simulink library "dspadpt3"  (Simulink 8.2)
settings: Solver=ode45  SolverMode=SingleTasking  StartTime=0.0  StopTime=10.0  RelTol=1e-3
values from neighbouring files (symbols this model uses):
  D = D + B    [rebuffer_delay.m]
undefined symbols (not defined in the file or in its folder): len_measure, len_state, num_cols, num_rows, param, slselsubs
libraries: dspsigattribs x12, dspmtrx3 x2, dspsigops x2, adptfiltsubsys x1, dspsolvers x1
settings Model: RequirementInfo=9  FPTRunName=Active  Creator=don  LastModifiedBy=sconahan  ExtModeAutoUpdateStatusClock=off
settings Model: ForwardingTableString=|
  | ||__slOldName__||dspadpt3/RLS
  | Adaptive Filter||__slNewName__||dspobslib/RLS
  | Adaptive Filter||__slOldName__||dspadpt3/LMS
  | Adaptive Filter||__slNewName__||dspobslib/LMS
  | Adaptive Filter||__slOldName__||dspadpt3/Kalman
  | Adaptive Filter||__slNewName__||dspobslib/Kalman
  | Adaptive Filter

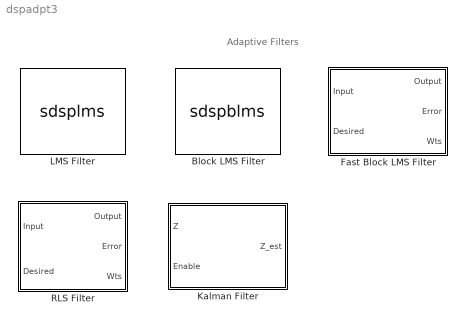
== system dspadpt3 ==
  note: Adaptive Filters
  Block LMS Filter : S-Function  FunctionName=sdspblms  Parameters=L,N,stepflag,mu,leakage,addnparflag,ic,Adapt,resetflag,weights  EnableBusSupport=off  mask(Block LMS Filter){algo=Block LMS, ShowPortLabels=off, L=32, N=32, stepflag=Dialog, mu=0.1, leakage=1.0, addnparflag=on, ic=0, Adapt=off, resetflag=None, weights=on}
      mask prompts: algo "dummy1"; ShowPortLabels "dummy2"; L "Filter length:"; N "Block size:"; stepflag "Specify step size via:"; mu "Step size (mu):"; leakage "Leakage factor (0 to 1):"; addnparflag "dummy3"; ic "Initial value of filter weights:"; Adapt "Adapt port"; resetflag "Reset port:"; weights "Output filter weights"
      mask help:
      | Computes filter weights based on the Block LMS algorithm for filtering of the input signal. The filter weights are updated once for every block of data that is processed.
      |
      | Select the Adapt port check box to create an Adapt port on the block. When the input to this port is nonzero, the block continuously updates the filter weights. When the input to this port is zero, the filter weights remain constant.
      |
      | If the Reset port is enabled and a reset event occurs, the block resets the filter weights to their initial values.
      mask init:
      | resetflag = resetflag-1;
      | [si,so]=dspblkblklms('icon');
      mask Help: eval('blocksethelp');
      mask TypeOptions algo: Block LMS | Fast Block LMS
      mask TypeOptions stepflag: Dialog | Input port
      mask Callback stepflag: dspblkblklms;
      mask TypeOptions resetflag: None | Rising edge | Falling edge | Either edge | Non-zero sample
      mask Display:
      | disp('Block\nLMS')
      | port_label('input',si(1).port, si(1).txt);
      | port_label('input',si(2).port, si(2).txt);
      | port_label('input',si(3).port, si(3).txt);
      | port_label('input',si(4).port, si(4).txt);
      | port_label('input',si(5).port, si(5).txt);
      | 
      | port_label('output',so(1).port, so(1).txt);
      | port_label('output',so(2).port, so(2).txt);
      | port_label('output',so(3).port, so(3).txt);
  Fast Block LMS Filter : Subsystem  mask(Fast Block LMS Filter){algo=Fast Block LMS, L=32, N=32, stepflag=Dialog, mu=0.008, leakage=1.0, addnparflag=on, ic=0, Adapt=off, resetflag=None, weights=on}
      mask prompts: algo "Algorithm:"; L "Filter length:"; N "Block size:"; stepflag "Specify step size via:"; mu "Step size (mu):"; leakage "Leakage factor (0 to 1):"; addnparflag "Dummy parameter"; ic "Initial value of filter weights:"; Adapt "Adapt port"; resetflag "Reset port:"; weights "Output filter weights"
      mask help:
      | Computes filter weights based on the Fast Block LMS algorithm for filtering of the input signal. The filter weights are updated once for every block of data that is processed. This block uses FFT for fast convolution.
      |
      | Select the Adapt port check box to create an Adapt port on the block. When the input to this port is nonzero, the block continuoulsy updates the filter weights. When the input to this port is zero, the filter weights remain constant.
      |
      | If the Reset port is enabled and a reset event occurs, the block resets the filter weights to their initial values.
      mask init:
      | dspblkfblms('init');
      settings: ErrorFcn=dspblkadpterrfcn
      mask Help: eval('blocksethelp');
      mask TypeOptions algo: Block LMS | Fast Block LMS
      mask TypeOptions stepflag: Dialog | Input port
      mask Callback stepflag: dspblkfblms('addparams');
      mask TypeOptions resetflag: None | Rising Edge | Falling Edge | Either Edge | Non-zero sample
      mask Display: disp('Fast Block\nLMS');
  Kalman Filter : Subsystem  DialogController=dspDDGCreate  DialogControllerArgs=DataTag0  mask(Kalman Filter){num_targets=10, sourceEnable=Specify via input port <Enable>, isReset=on, X=zeros([6, 1]), P=10*eye(6), A=[1 0 1 0 0 0;0 1 0 1 0 0; 0 0 1 0 0 0; 0 0 0 1 0 0; 0 0 0 0 1 0; 0 0 0 0 0 1], sourceMeasure=Specify via Dialog, H=[1 0 0 0 0 0; 0 1 0 0 0 0; 0 0 0 0 1 0; 0 0 0 0 0 1], Q=0.05*eye(6), R=eye(4), isOutputEstMeasure=on, isOutputEstState=off, isOutputEstError=off, isOutputPrdMeasure=off, isOutputPrdState=off, isOutputPrdError=off}
      mask prompts: num_targets "Number of filters:"; sourceEnable "Enable filters:"; isReset "Reset estimated state and estimated error covariance when filters are disabled"; X "Initial condition for state:"; P "Initial condition for estimation error covariance:"; A "State transition matrix:"; sourceMeasure "Measurement matrix source:"; H "Measurement matrix:"; Q "Process noise covariance:"; R "Measurement noise covariance:"; isOutputEstMeasure "Output updated measurement"; isOutputEstState "Output updated state"; isOutputEstError "Output updated estimation error"; isOutputPrdMeasure "Output predicted measurement"; isOutputPrdState "Output predicted state"; isOutputPrdError "Output predicted estimation error"
      mask help:
      | Estimate the state of a dynamic system from a series of incomplete and/or noisy measurements. This block can use the previously estimated state to predict the current state. It can also use the current measurement and the predicted state to estimate the current state value.
      |
      | All filters have the same state transition matrix, measurement matrix, initial conditions, and noise covariance, but their state, measurement, enable, and MSE signals are unique. Within the state, measurement, enable, and MSE signals, each column corresponds to a filter.
      mask init:
      | blkh = gcbh;
      | [len_state,len_measure,param] = deal(1,1,[]);
      | % Check for the presence of at least one output port and reconfigure block based on control parameters
      | errmsg = dspblkkalman('init',blkh,sourceEnable,isReset,sourceMeasure,isOutputEstMeasure,isOutputEstState,isOutputEstError,isOutputPrdMeasure,isOutputPrdState,isOutputPrdError);
      | % Get names for existing ports
      | [inport,outport] = dspblkkalman('icon', blkh);
      | if isempty(errmsg)
      |     % Check remaining parameters. Some checking was already done, by the dialog callback and by the above call to dspblkkalman.
      |     [errmsg,num_targets,len_state,len_measure,param] = dspblkkalman('check_param',blkh,true,sourceMeasure,num_targets,A,H,X,P,R,Q);
      | end
      | if ~isempty(errmsg)
      |     error(errmsg);
      | end
      mask Help: eval('blocksethelp');
      mask TypeOptions sourceEnable: Always | Specify via input port <Enable>
      mask TypeOptions sourceMeasure: Specify via Dialog | Input port <H>
      mask Display:
      | disp('Kalman\nFilter');
      | port_label('input',1, 'Z');
      | port_label('input',inport(1).port, inport(1).txt);
      | port_label('input',inport(2).port, inport(2).txt);
      | port_label('output',outport(1).port, outport(1).txt);
      | port_label('output',outport(2).port, outport(2).txt);
      | port_label('output',outport(3).port, outport(3).txt);
      | port_label('output',outport(4).port, outport(4).txt);
      | port_label('output',outport(5).port, outport(5).txt);
      | port_label('output',outport(6).port, outport(6).txt);
  LMS Filter : S-Function  DialogController=dspDDGCreate  DialogControllerArgs=DataTag1  FunctionName=sdsplms  Parameters=Algo,L,stepflag,mu,leakage,ic,Adapt,resetflag,weights,dtInfo.firstCoeffMode,dtInfo.firstCoeffWordLength,dtInfo.firstCoeffFracLength,dtInfo.secondCoeffMode,dtInfo.secondCoeffWordLength,dtInfo.secondCoeffFracLength,dtInfo.prodOutputMode,dtInfo.prodOutputWordLength,dtInfo.prodOutputFracLength,dtInfo.prodOutput2Mode,dtInfo.prodOutput2WordLength,dtInfo.prodOutput2FracLength,dtInfo.prodOutput3Mode,dtInfo.prodOutput3WordLength,dtInfo.prodOutput3FracLength,dtInfo.prodOutput4Mode,dtInfo.prodOutput4WordLength,dtInfo.prodOutput4FracLength,dtInfo.quotientMode,dtInfo.quotientWordLength,dtInfo.quotientFracLength,dtInfo.accumMode,dtInfo.accumWordLength,dtInfo.accumFracLength,dtInfo.accum2Mode,dtInfo.accum2WordLength,dtInfo.accum2FracLength,dtInfo.memoryMode,dtInfo.memoryWordLength,dtInfo.memoryFracLength,dtInfo.roundingMode,dtInfo.overflowMode  EnableBusSupport=off  mask(LMS Filter){ShowPortLabels=off, Algo=LMS, L=32, stepflag=Dialog, mu=0.1, leakage=1.0, ic=0, Adapt=off, resetflag=None, weights=on, firstCoeffMode=Same word length as first input, firstCoeffWordLength=16, firstCoeffFracLength=15, secondCoeffMode=User-defined, secondCoeffWordLength=2, secondCoeffFracLength=15, accumMode=Same as first input, accumWordLength=32, accumFracLength=20, accum2Mode=User-defined, accum2FracLength=20, prodOutputMode=Same as first input, prodOutputWordLength=32, prodOutputFracLength=20, prodOutput2Mode=User-defined, prodOutput2FracLength=20, prodOutput3Mode=User-defined, prodOutput3FracLength=20, prodOutput4Mode=User-defined, prodOutput4FracLength=20, quotientMode=User-defined, quotientFracLength=20, memoryMode=Same as first input, memoryWordLength=16, memoryFracLength=15, roundingMode=Floor, overflowMode=off, addnparflag=off, LockScale=off}
      mask prompts: ShowPortLabels "dummy"; Algo "Algorithm:"; L "Filter length:"; stepflag "Specify step size via:"; mu "Step size (mu):"; leakage "Leakage factor (0 to 1):"; ic "Initial value of filter weights:"; Adapt "Adapt port"; resetflag "Reset port:"; weights "Output filter weights"; firstCoeffMode "Step size (mu) attributes:"; firstCoeffWordLength "Step size (mu) word length:"; firstCoeffFracLength "Step size (mu) fraction length:"; secondCoeffMode "Leakage factor attributes:"; secondCoeffWordLength "DUMMY lkg wordlength:"; secondCoeffFracLength "Leakage factor fraction length:"; accumMode "Accumulator (XTX) attributes:"; accumWordLength "Accumulator (XTX) word length:"; accumFracLength "Accumulator (XTX) fraction length:"; accum2Mode "Accumulator (WTX) attributes:"; accum2FracLength "Accumulator (WTX) fraction length:"; prodOutputMode "Product (XTX) output attributes:"; prodOutputWordLength "Product (XTX) output word length:"; prodOutputFracLength "Product (XTX) output fraction length:"; prodOutput2Mode "Product (WTX) output attributes:"; prodOutput2FracLength "Product (WTX) output fraction length:"; prodOutput3Mode "Product (mu*e) output attributes:"; prodOutput3FracLength "Product (mu*e) output fraction length:"; prodOutput4Mode "Product (Q*x) output attributes:"; prodOutput4FracLength "Product (Q*x) output fraction length:"; quotientMode "Quotient attributes:"; quotientFracLength "Quotient fraction length:"; memoryMode "State memory attributes:"; memoryWordLength "State memory word length:"; memoryFracLength "State memory fraction length:"; roundingMode "Round integer calculations toward:"; overflowMode "Saturate on integer overflow"; addnparflag "Dummy parameter"; LockScale "Lock scaling"
      mask help:
      | Adapts the filter weights based on the chosen algorithm for filtering of the input signal.
      |
      | Select the Adapt port check box to create an Adapt port on the block. When the input to this port is nonzero, the block continuously updates the filter weights. When the input to this port is zero, the filter weights remain constant.
      |
      | If the Reset port is enabled and a reset event occurs, the block resets the filter weights to their initial values.
      mask init:
      | resetflag = resetflag-1;
      | ic        = flipud(ic(:));
      | dtInfo    = dspblkGetLMSFilterDTRowInfo(gcbh);
      | [si,so,disp_str] = dspblklms;
      mask Help: eval('blocksethelp');
      mask TypeOptions Algo: LMS | Normalized LMS | Sign-Error LMS | Sign-Data LMS | Sign-Sign LMS
      mask TypeOptions stepflag: Dialog | Input port
      mask TypeOptions resetflag: None | Rising edge | Falling edge | Either edge | Non-zero sample
      mask TypeOptions firstCoeffMode: Same word length as first input | Specify word length | Binary point scaling | Slope and bias scaling | User-defined
      mask TypeOptions secondCoeffMode: Same word length as first input | Specify word length | Binary point scaling | Slope and bias scaling | User-defined
      mask TypeOptions accumMode: Same as first input | Binary point scaling | Slope and bias scaling | User-defined
      mask TypeOptions accum2Mode: Same as first accumulator | Binary point scaling | Slope and bias scaling | User-defined
      mask TypeOptions prodOutputMode: Same as first input | Binary point scaling | Slope and bias scaling | User-defined
      mask TypeOptions prodOutput2Mode: Same as first product | Binary point scaling | Slope and bias scaling | User-defined
      mask TypeOptions prodOutput3Mode: Same as first product | Binary point scaling | Slope and bias scaling | User-defined
      mask TypeOptions prodOutput4Mode: Same as first product | Binary point scaling | Slope and bias scaling | User-defined
      mask TypeOptions quotientMode: Same as first product | Binary point scaling | Slope and bias scaling | User-defined
      mask TypeOptions memoryMode: Same as first input | Binary point scaling | Slope and bias scaling | User-defined
      mask TypeOptions roundingMode: Ceiling | Convergent | Floor | Nearest | Round | Simplest | Zero
      mask Display:
      | disp(disp_str)
      | port_label('input',si(1).port, si(1).txt);
      | port_label('input',si(2).port, si(2).txt);
      | port_label('input',si(3).port, si(3).txt);
      | port_label('input',si(4).port, si(4).txt);
      | port_label('input',si(5).port, si(5).txt);
      | 
      | port_label('output',so(1).port, so(1).txt);
      | port_label('output',so(2).port, so(2).txt);
      | port_label('output',so(3).port, so(3).txt);
  RLS Filter : Subsystem  mask(RLS filter){L=32, lambdaflag=Dialog, lambda=1.0, addnparflag=on, ic=0, delta=0.1, Adapt=off, resetflag=None, weights=on}
      mask prompts: L "Filter length:"; lambdaflag "Specify forgetting factor via:"; lambda "Forgetting factor (0 to 1):"; addnparflag "Dummy parameter"; ic "Initial value of filter weights:"; delta "Initial input variance estimate:"; Adapt "Adapt port"; resetflag "Reset port:"; weights "Output filter weights"
      mask help:
      | Computes filter weights based on the exponentially weighted recursive least-squares (RLS) algorithm for adaptive filtering of the input signal.
      |
      | Select the Adapt port check box to create an Adapt port on the block. When the input to this port is nonzero, the block continuoulsy updates the filter weights. When the input to this port is zero, the filter weights remain constant.
      |
      | If the Reset port is enabled and a reset event occurs, the block resets the filter weights to their initial values.
      mask init:
      | dspblkrls('init', L, lambda, ic);
      settings: ErrorFcn=dspblkadpterrfcn
      mask Help: eval('blocksethelp');
      mask TypeOptions lambdaflag: Dialog | Input port
      mask Callback lambdaflag: dspblkrls('addparams');
      mask TypeOptions resetflag: None | Rising edge | Falling edge | Either edge | Non-zero sample
      mask Display: disp('RLS');

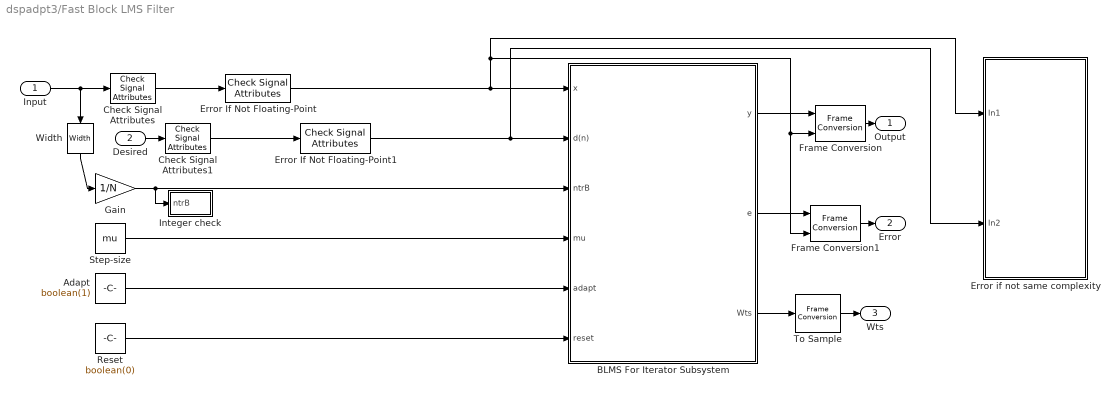
== system dspadpt3/Fast Block LMS Filter ==
  Input : Inport
  Desired : Inport  Port=2
  Adapt : Constant  Value=boolean(1)
  BLMS For Iterator Subsystem : Subsystem  TreatAsAtomicUnit=on  mask{algo_for=Fast Block LMS, stepflag_for=off, weights_for=on}
      mask prompts: algo_for "Algorithm:"; stepflag_for "Input step size via port:"; weights_for "Send filter weights to output:"
      mask init:
      | dspblkfblmsfor;
      mask TypeOptions algo_for: Block LMS | Fast Block LMS
  Check Signal Attributes : dspsigattribs/Check Signal Attributes  SigAttribCheckMethod=Matches attributes exactly  Complexity=Ignore  Frame=Ignore  DimsCheckMethod=Is...  Dimensions=Full matrix (2-D)  DatatypeCheckMethod=Ignore  DatatypeGeneral=Boolean  DtypeFloatSpecific=Any floating-point  DtypeFixedSpecific=Any fixed-point  DtypeIntSpecific=Any integer  SampleMode=Ignore
  Check Signal Attributes1 : dspsigattribs/Check Signal Attributes  SigAttribCheckMethod=Matches attributes exactly  Complexity=Ignore  Frame=Ignore  DimsCheckMethod=Is...  Dimensions=Full matrix (2-D)  DatatypeCheckMethod=Ignore  DatatypeGeneral=Boolean  DtypeFloatSpecific=Any floating-point  DtypeFixedSpecific=Any fixed-point  DtypeIntSpecific=Any integer  SampleMode=Ignore
  Error If Not Floating-Point : dspsigattribs/Check Signal Attributes  SigAttribCheckMethod=Does not match attributes exactly  Complexity=Ignore  Frame=Ignore  DimsCheckMethod=Ignore  Dimensions=1-D  DatatypeCheckMethod=Is...  DatatypeGeneral=Floating-point  DtypeFloatSpecific=Any floating-point  DtypeFixedSpecific=Any fixed-point  DtypeIntSpecific=Any integer  SampleMode=Ignore
  Error If Not Floating-Point1 : dspsigattribs/Check Signal Attributes  SigAttribCheckMethod=Does not match attributes exactly  Complexity=Ignore  Frame=Ignore  DimsCheckMethod=Ignore  Dimensions=1-D  DatatypeCheckMethod=Is...  DatatypeGeneral=Floating-point  DtypeFloatSpecific=Any floating-point  DtypeFixedSpecific=Any fixed-point  DtypeIntSpecific=Any integer  SampleMode=Ignore
  Error if not same complexity : Subsystem  TreatAsAtomicUnit=on  SimViewingDevice=on
  Frame Conversion : FrameConversion  InheritSamplingMode=on
  Frame Conversion1 : FrameConversion  InheritSamplingMode=on
  Gain : Gain  Gain=1/N  SaturateOnIntegerOverflow=on  OutDataTypeStr=Inherit: Same as input  ParamDataTypeStr=Inherit: Same as input
  Integer check : Subsystem
  Reset : Constant  Value=boolean(0)
  Step-size : Constant  Value=mu  OutDataTypeStr=Inherit: Inherit via back propagation
  To Sample : FrameConversion  OutFrame=Sample-based
  Width : Width
  Output : Outport
  Error : Outport  Port=2
  Wts : Outport  Port=3
  wires:
  Step-size/1 -> BLMS For Iterator Subsystem/4(mu)
  To Sample/1 -> Wts/1
  BLMS For Iterator Subsystem/3(Wts) -> To Sample/1
  Desired/1 -> Check Signal Attributes1/1
  Input/1 -> Width/1, Check Signal Attributes/1
  Gain/1 -> Integer check/1(ntrB), BLMS For Iterator Subsystem/3(ntrB)
  Width/1 -> Gain/1
  Reset/1 -> BLMS For Iterator Subsystem/6(reset)
  Adapt/1 -> BLMS For Iterator Subsystem/5(adapt)
  BLMS For Iterator Subsystem/1(y) -> Frame Conversion/1
  Frame Conversion/1 -> Output/1
  BLMS For Iterator Subsystem/2(e) -> Frame Conversion1/1
  Frame Conversion1/1 -> Error/1
  Error If Not Floating-Point/1 -> Frame Conversion/2, Frame Conversion1/2, Error if not same complexity/1(In1), BLMS For Iterator Subsystem/1(x)
  Error If Not Floating-Point1/1 -> Error if not same complexity/2(In2), BLMS For Iterator Subsystem/2(d(n))
  Check Signal Attributes1/1 -> Error If Not Floating-Point1/1
  Check Signal Attributes/1 -> Error If Not Floating-Point/1

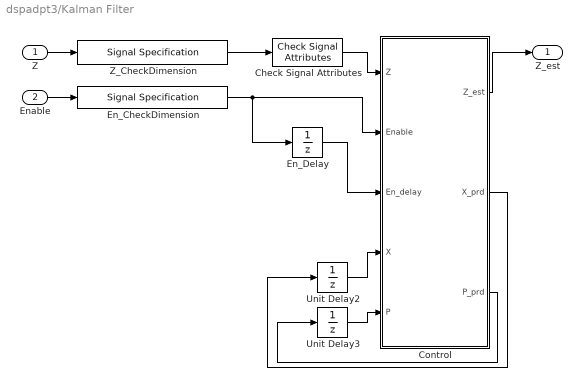
== system dspadpt3/Kalman Filter ==
  Z : Inport
  Enable : Inport  Port=2
  Check Signal Attributes : dspsigattribs/Check Signal Attributes  SigAttribCheckMethod=Does not match attributes exactly  Complexity=Real  Frame=Ignore  DimsCheckMethod=Ignore  Dimensions=Scalar (1-D or 2-D)  DatatypeCheckMethod=Is...  DatatypeGeneral=Floating-point  DtypeFloatSpecific=Any floating-point  DtypeFixedSpecific=Any fixed-point  DtypeIntSpecific=Any integer  SampleMode=Ignore
  Control : Subsystem
  En_CheckDimension : SignalSpecification  Dimensions=[1, num_targets]
  En_Delay : UnitDelay  SampleTime=-1
  Unit Delay2 : UnitDelay  InitialCondition=param.XAll  SampleTime=-1
  Unit Delay3 : UnitDelay  InitialCondition=param.PAll  SampleTime=-1
  Z_CheckDimension : SignalSpecification  Dimensions=[len_measure, num_targets]
  Z_est : Outport
  wires:
  Unit Delay2/1 -> Control/4(X)
  Unit Delay3/1 -> Control/5(P)
  Z_CheckDimension/1 -> Check Signal Attributes/1
  Z/1 -> Z_CheckDimension/1
  Control/1(Z_est) -> Z_est/1
  Check Signal Attributes/1 -> Control/1(Z)
  Control/2(X_prd) -> Unit Delay2/1
  Control/3(P_prd) -> Unit Delay3/1
  Enable/1 -> En_CheckDimension/1
  En_CheckDimension/1 -> En_Delay/1, Control/2(Enable)
  En_Delay/1 -> Control/3(En_delay)

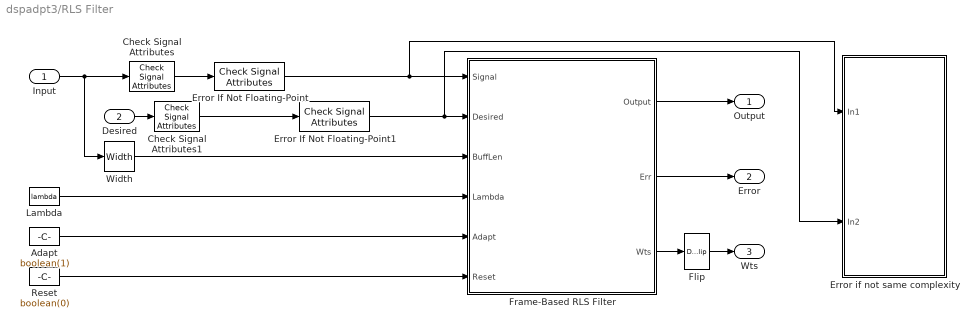
== system dspadpt3/RLS Filter ==
  Input : Inport
  Desired : Inport  Port=2
  Adapt : Constant  Value=boolean(1)
  Check Signal Attributes : dspsigattribs/Check Signal Attributes  SigAttribCheckMethod=Matches attributes exactly  Complexity=Ignore  Frame=Ignore  DimsCheckMethod=Is...  Dimensions=Full matrix (2-D)  DatatypeCheckMethod=Ignore  DatatypeGeneral=Boolean  DtypeFloatSpecific=Any floating-point  DtypeFixedSpecific=Any fixed-point  DtypeIntSpecific=Any integer  SampleMode=Ignore
  Check Signal Attributes1 : dspsigattribs/Check Signal Attributes  SigAttribCheckMethod=Matches attributes exactly  Complexity=Ignore  Frame=Ignore  DimsCheckMethod=Is...  Dimensions=Full matrix (2-D)  DatatypeCheckMethod=Ignore  DatatypeGeneral=Boolean  DtypeFloatSpecific=Any floating-point  DtypeFixedSpecific=Any fixed-point  DtypeIntSpecific=Any integer  SampleMode=Ignore
  Error If Not Floating-Point : dspsigattribs/Check Signal Attributes  SigAttribCheckMethod=Does not match attributes exactly  Complexity=Ignore  Frame=Ignore  DimsCheckMethod=Ignore  Dimensions=1-D  DatatypeCheckMethod=Is...  DatatypeGeneral=Floating-point  DtypeFloatSpecific=Any floating-point  DtypeFixedSpecific=Any fixed-point  DtypeIntSpecific=Any integer  SampleMode=Ignore
  Error If Not Floating-Point1 : dspsigattribs/Check Signal Attributes  SigAttribCheckMethod=Does not match attributes exactly  Complexity=Ignore  Frame=Ignore  DimsCheckMethod=Ignore  Dimensions=1-D  DatatypeCheckMethod=Is...  DatatypeGeneral=Floating-point  DtypeFloatSpecific=Any floating-point  DtypeFixedSpecific=Any fixed-point  DtypeIntSpecific=Any integer  SampleMode=Ignore
  Error if not same complexity : Subsystem  TreatAsAtomicUnit=on  SimViewingDevice=on
  Flip : DSPFlip
  Frame-Based RLS Filter : Subsystem  TreatAsAtomicUnit=on  mask{weights_for=on}
      mask prompts: weights_for "Send filter weights to output:"
      mask init:
      | dspblkrlsfor;
  Lambda : Constant  Value=lambda  OutDataTypeStr=Inherit: Inherit via back propagation
  Reset : Constant  Value=boolean(0)
  Width : Width
  Output : Outport
  Error : Outport  Port=2
  Wts : Outport  Port=3
  wires:
  Check Signal Attributes/1 -> Error If Not Floating-Point/1
  Error If Not Floating-Point1/1 -> Error if not same complexity/2(In2), Frame-Based RLS Filter/2(Desired)
  Error If Not Floating-Point/1 -> Error if not same complexity/1(In1), Frame-Based RLS Filter/1(Signal)
  Check Signal Attributes1/1 -> Error If Not Floating-Point1/1
  Lambda/1 -> Frame-Based RLS Filter/4(Lambda)
  Adapt/1 -> Frame-Based RLS Filter/5(Adapt)
  Width/1 -> Frame-Based RLS Filter/3(BuffLen)
  Input/1 -> Check Signal Attributes/1, Width/1
  Desired/1 -> Check Signal Attributes1/1
  Frame-Based RLS Filter/1(Output) -> Output/1
  Reset/1 -> Frame-Based RLS Filter/6(Reset)
  Frame-Based RLS Filter/2(Err) -> Error/1
  Frame-Based RLS Filter/3(Wts) -> Flip/1
  Flip/1 -> Wts/1

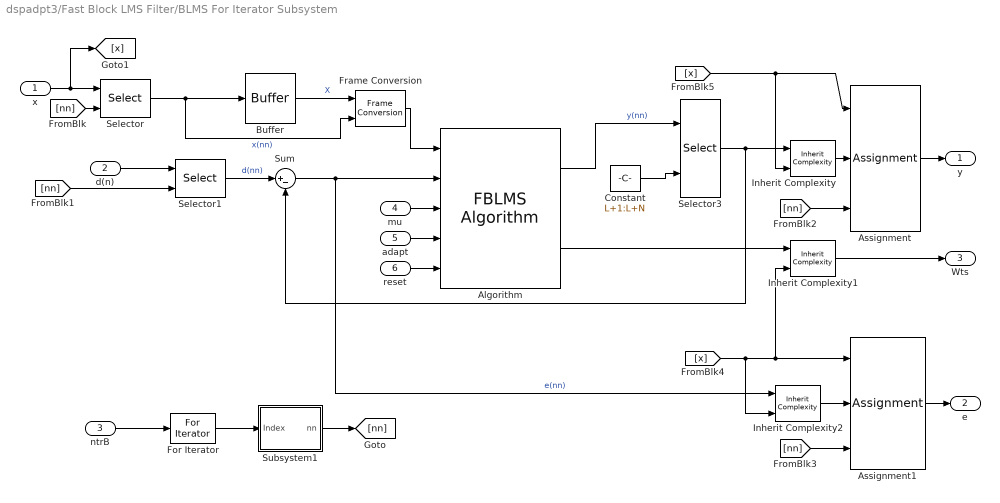
== system dspadpt3/Fast Block LMS Filter/BLMS For Iterator Subsystem ==
  x : Inport
  d(n) : Inport  Port=2
  ntrB : Inport  Port=3
  mu : Inport  Port=4
  adapt : Inport  Port=5
  reset : Inport  Port=6
  Algorithm : adptfiltsubsys/FBLMS Algorithm  weights_algo=on
  Assignment : Assignment  IndexOptions=Index vector (port)  Indices=1  OutputSizes=[1 1]
  Assignment1 : Assignment  IndexOptions=Index vector (port)  Indices=1  OutputSizes=[1 1]
  Buffer : Buffer  N=L+N  V=L  TreatMby1Signals=One channel
  Constant : Constant  Value=L+1:L+N
  For Iterator : ForIterator  IterationSource=external  IterationVariableDataType=double
  Frame Conversion : FrameConversion  InheritSamplingMode=on
  Inherit Complexity : dspsigattribs/Inherit Complexity
  Inherit Complexity1 : dspsigattribs/Inherit Complexity
  Inherit Complexity2 : dspsigattribs/Inherit Complexity
  Selector : Selector  IndexOptions=Index vector (port)  Indices=[1 3]  OutputSizes=1
  Selector1 : Selector  IndexOptions=Index vector (port)  Indices=[1 3]  OutputSizes=1
  Selector3 : Selector  IndexOptions=Index vector (port)  Indices=[1 3]  OutputSizes=1
  Subsystem1 : Subsystem
  Sum : Sum  Inputs=|+-  SaturateOnIntegerOverflow=on
  y : Outport
  e : Outport  Port=2
  Wts : Outport  Port=3
  wires:
  Algorithm/2 -> Inherit Complexity1/1
  adapt/1 -> Algorithm/4
  mu/1 -> Algorithm/3
  Inherit Complexity1/1 -> Wts/1
  Inherit Complexity2/1 -> Assignment1/2
  Inherit Complexity/1 -> Assignment/2
  Sum/1 -> Algorithm/2, Inherit Complexity2/1  "e(nn)"
  Selector1/1 -> Sum/1  "d(nn)"
  [nn] -> Assignment1/3
  Assignment1/1 -> e/1
  ntrB/1 -> For Iterator/1
  For Iterator/1 -> Subsystem1/1(Index)
  Assignment/1 -> y/1
  x/1 -> Selector/1, [x]
  [nn] -> Selector/2
  d(n)/1 -> Selector1/1
  [nn] -> Selector1/2
  Subsystem1/1(nn) -> [nn]
  Selector/1 -> Frame Conversion/2, Buffer/1  "x(nn)"
  reset/1 -> Algorithm/5
  Constant/1 -> Selector3/2
  Selector3/1 -> Sum/2, Inherit Complexity/1
  Algorithm/1 -> Selector3/1  "y(nn)"
  [nn] -> Assignment/3
  [x] -> Inherit Complexity2/2, Assignment1/1, Inherit Complexity1/2
  [x] -> Inherit Complexity/2, Assignment/1
  Buffer/1 -> Frame Conversion/1  "X"
  Frame Conversion/1 -> Algorithm/1

== system dspadpt3/Fast Block LMS Filter/Error if not same complexity ==
  In1 : Inport
  In2 : Inport  Port=2
  Assertion : Assertion  AssertionFailFcn=error('The signals connected to the Input and Desired ports of the Fast Block LMS Filter block must have the same complexity.')
  Probe : Probe  ProbeWidth=off  ProbeSampleTime=off  ProbeComplexityDataType=boolean
  Probe1 : Probe  ProbeWidth=off  ProbeSampleTime=off  ProbeComplexityDataType=boolean
  Relational Operator : RelationalOperator  Operator===  OutDataTypeStr=boolean  ZeroCross=off  InputSameDT=on
  wires:
  Relational Operator/1 -> Assertion/1
  In2/1 -> Probe1/1
  In1/1 -> Probe/1
  Probe1/1 -> Relational Operator/2
  Probe/1 -> Relational Operator/1

== system dspadpt3/Fast Block LMS Filter/Integer check ==
  ntrB : Inport
  Assertion : Assertion  AssertionFailFcn=error('The input frame length is not an integer multiple of the Block length');
  Relational Operator : RelationalOperator  Operator===  OutDataTypeStr=boolean
  Rounding Function : Rounding  Operator=fix
  wires:
  Rounding Function/1 -> Relational Operator/2
  Relational Operator/1 -> Assertion/1
  ntrB/1 -> Relational Operator/1, Rounding Function/1

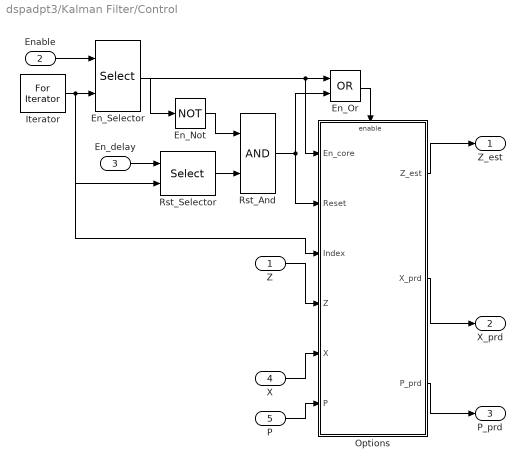
== system dspadpt3/Kalman Filter/Control ==
  Z : Inport
  Enable : Inport  Port=2
  En_delay : Inport  Port=3
  X : Inport  Port=4
  P : Inport  Port=5
  En_Not : Logic  Operator=NOT  AllPortsSameDT=off
  En_Or : Logic  Operator=OR  AllPortsSameDT=off
  En_Selector : Selector  NumberOfDimensions=2  IndexOptions=Select all,Index vector (port)  Indices=-1,1  OutputSizes=1
  Iterator : ForIterator  IterationLimit=num_targets
  Options : Subsystem
  Rst_And : Logic  AllPortsSameDT=off
  Rst_Selector : Selector  NumberOfDimensions=2  IndexOptions=Select all,Index vector (port)  Indices=-1,1  OutputSizes=1
  Z_est : Outport
  X_prd : Outport  Port=2
  P_prd : Outport  Port=3
  wires:
  Iterator/1 -> Options/3(Index), En_Selector/2, Rst_Selector/2
  Options/1(Z_est) -> Z_est/1
  Options/2(X_prd) -> X_prd/1
  Options/3(P_prd) -> P_prd/1
  Z/1 -> Options/4(Z)
  X/1 -> Options/5(X)
  P/1 -> Options/6(P)
  Enable/1 -> En_Selector/1
  En_delay/1 -> Rst_Selector/1
  En_Selector/1 -> En_Not/1, En_Or/1, Options/1(En_core)
  En_Not/1 -> Rst_And/1
  Rst_Selector/1 -> Rst_And/2
  Rst_And/1 -> En_Or/2, Options/2(Reset)
  En_Or/1 -> Options/Enable

== system dspadpt3/RLS Filter/Error if not same complexity ==
  In1 : Inport
  In2 : Inport  Port=2
  Assertion : Assertion  AssertionFailFcn=error('The signals connected to the Input and Desired ports of the RLS Filter block must have the same complexity.')
  Probe : Probe  ProbeWidth=off  ProbeSampleTime=off  ProbeComplexityDataType=boolean
  Probe1 : Probe  ProbeWidth=off  ProbeSampleTime=off  ProbeComplexityDataType=boolean
  Relational Operator : RelationalOperator  Operator===  OutDataTypeStr=boolean  ZeroCross=off  InputSameDT=on
  wires:
  Relational Operator/1 -> Assertion/1
  In2/1 -> Probe1/1
  In1/1 -> Probe/1
  Probe1/1 -> Relational Operator/2
  Probe/1 -> Relational Operator/1

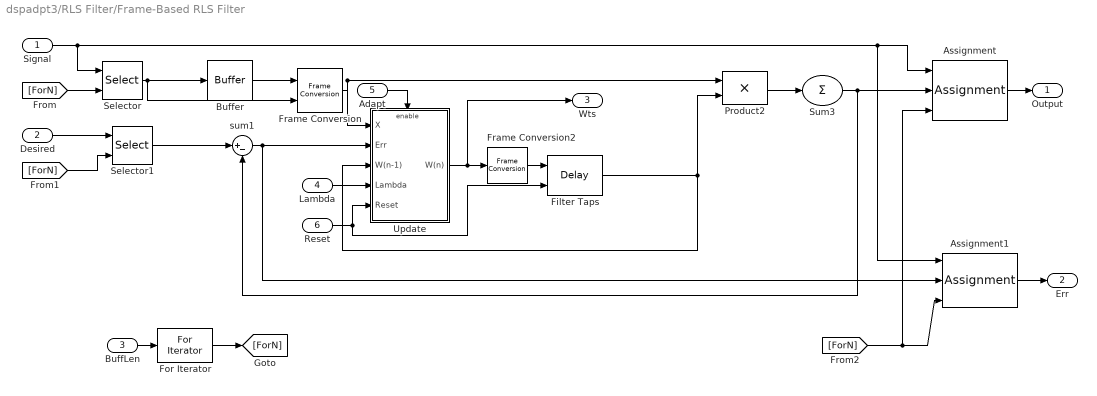
== system dspadpt3/RLS Filter/Frame-Based RLS Filter ==
  Signal : Inport
  Desired : Inport  Port=2
  BuffLen : Inport  Port=3
  Lambda : Inport  Port=4
  Adapt : Inport  Port=5
  Reset : Inport  Port=6
  Assignment : Assignment  IndexOptions=Index vector (port)  Indices=1  OutputSizes=[1 1]
  Assignment1 : Assignment  IndexOptions=Index vector (port)  Indices=1  OutputSizes=[1 1]
  Buffer : Buffer  N=L  V=L-1  TreatMby1Signals=One channel
  Filter Taps : dspsigops/Delay  dly_unit=Samples  delay=1  ic_detail=on  dif_ic_for_ch=off  dif_ic_for_dly=off  ic=flipud(ic(:))  reset_popup=Non-zero sample
  For Iterator : ForIterator  IterationSource=external  IterationLimit=4
  Frame Conversion : FrameConversion  InheritSamplingMode=on
  Frame Conversion2 : FrameConversion  OutFrame=Sample-based
  Product2 : Product  SaturateOnIntegerOverflow=on  OutDataTypeStr=Inherit: Same as first input
  Selector : Selector  IndexOptions=Index vector (port)  Indices=[1 3]  OutputSizes=1
  Selector1 : Selector  IndexOptions=Index vector (port)  Indices=[1 3]  OutputSizes=1
  Sum3 : Sum  Inputs=1  SaturateOnIntegerOverflow=on
  Update : Subsystem
  sum1 : Sum  Inputs=|+-  SaturateOnIntegerOverflow=on  InputSameDT=on  OutDataTypeStr=Inherit: Same as first input
  Output : Outport
  Err : Outport  Port=2
  Wts : Outport  Port=3
  wires:
  Frame Conversion/1 -> Update/1(X), Product2/1
  Lambda/1 -> Update/4(Lambda)
  Adapt/1 -> Update/Enable
  [ForN] -> Assignment1/3, Assignment/3
  Reset/1 -> Update/5(Reset), Filter Taps/2
  sum1/1 -> Assignment1/2, Update/2(Err)
  Sum3/1 -> Assignment/2, sum1/2
  Product2/1 -> Sum3/1
  Update/1(W(n)) -> Wts/1, Frame Conversion2/1
  Buffer/1 -> Frame Conversion/1
  Signal/1 -> Assignment1/1, Assignment/1, Selector/1
  Assignment/1 -> Output/1
  Desired/1 -> Selector1/1
  BuffLen/1 -> For Iterator/1
  Selector/1 -> Frame Conversion/2, Buffer/1
  For Iterator/1 -> [ForN]
  [ForN] -> Selector/2
  [ForN] -> Selector1/2
  Selector1/1 -> sum1/1
  Assignment1/1 -> Err/1
  Frame Conversion2/1 -> Filter Taps/1
  Filter Taps/1 -> Product2/2, Update/3(W(n-1))

== system dspadpt3/Fast Block LMS Filter/BLMS For Iterator Subsystem/Subsystem1 ==
  Index : Inport
  BlkVec : Constant  Value=[1:N]
  Constant : Constant
  Gain : Gain  Gain=N  SaturateOnIntegerOverflow=on  OutDataTypeStr=Inherit: Same as input  ParamDataTypeStr=Inherit: Same as input
  Sum : Sum  Inputs=|+-  SaturateOnIntegerOverflow=on
  Sum1 : Sum  Inputs=|++  SaturateOnIntegerOverflow=on
  nn : Outport
  wires:
  Sum1/1 -> nn/1
  Index/1 -> Sum/1  "n"
  BlkVec/1 -> Sum1/2  "i"
  Gain/1 -> Sum1/1  "(n-1)*N"
  Sum/1 -> Gain/1  "n-1"
  Constant/1 -> Sum/2

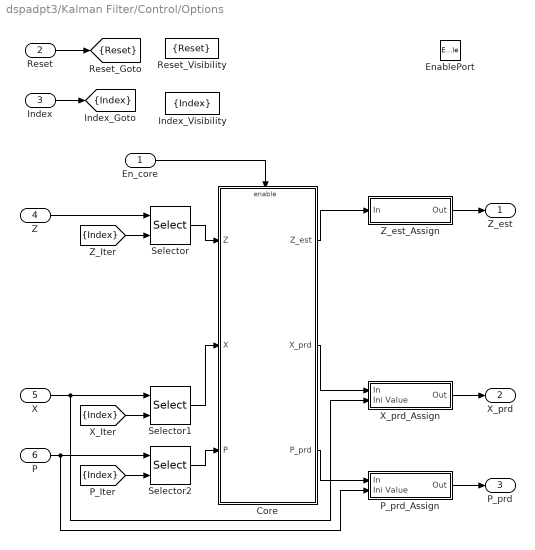
== system dspadpt3/Kalman Filter/Control/Options ==
  En_core : Inport
  Reset : Inport  Port=2
  Index : Inport  Port=3
  Z : Inport  Port=4
  X : Inport  Port=5
  P : Inport  Port=6
  EnablePort : EnablePort
  Core : Subsystem
  Index_Visibility : GotoTagVisibility  GotoTag=Index
  P_prd_Assign : Subsystem
  Reset_Visibility : GotoTagVisibility  GotoTag=Reset
  Selector : Selector  NumberOfDimensions=2  InputPortWidth=3  IndexOptions=Select all,Index vector (port)  Indices=-1,1  OutputSizes=1
  Selector1 : Selector  NumberOfDimensions=2  InputPortWidth=3  IndexOptions=Select all,Index vector (port)  Indices=-1,1  OutputSizes=1
  Selector2 : Selector  NumberOfDimensions=2  InputPortWidth=3  IndexOptions=Select all,Index vector (port)  Indices=-1,1  OutputSizes=1
  X_prd_Assign : Subsystem
  Z_est_Assign : Subsystem  mask{reset_value=zeros(len_measure, 1), num_rows=len_measure, num_cols=num_targets}
      mask prompts: reset_value "Default values:"; num_rows "Number of rows:"; num_cols "Number of Columns:"
      mask Display: disp('Assign/reset')
  Z_est : Outport
  X_prd : Outport  Port=2
  P_prd : Outport  Port=3
  tag scope: Index=scoped, Reset=scoped
  wires:
  Selector/1 -> Core/1(Z)
  X/1 -> Selector1/1, X_prd_Assign/2(Ini Value)
  [Index] -> Selector/2
  [Index] -> Selector2/2
  [Index] -> Selector1/2
  P/1 -> Selector2/1, P_prd_Assign/2(Ini Value)
  Z/1 -> Selector/1
  Selector1/1 -> Core/2(X)
  Selector2/1 -> Core/3(P)
  Core/2(X_prd) -> X_prd_Assign/1(In)
  X_prd_Assign/1(Out) -> X_prd/1
  Core/1(Z_est) -> Z_est_Assign/1(In)
  Core/3(P_prd) -> P_prd_Assign/1(In)
  Z_est_Assign/1(Out) -> Z_est/1
  P_prd_Assign/1(Out) -> P_prd/1
  Index/1 -> [Index]
  Reset/1 -> [Reset]
  En_core/1 -> Core/Enable

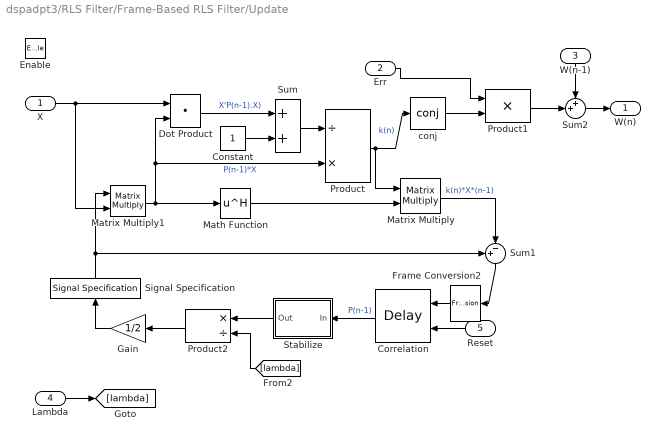
== system dspadpt3/RLS Filter/Frame-Based RLS Filter/Update ==
  X : Inport
  Err : Inport  Port=2
  W(n-1) : Inport  Port=3
  Lambda : Inport  Port=4
  Reset : Inport  Port=5
  Enable : EnablePort
  Constant : Constant  OutDataTypeStr=Inherit: Inherit via back propagation
  Correlation : dspsigops/Delay  dly_unit=Samples  delay=1  ic_detail=on  dif_ic_for_ch=on  dif_ic_for_dly=off  ic=eye(L)./delta  reset_popup=Non-zero sample
  Dot Product : DotProduct  InputSameDT=on  OutDataTypeStr=Inherit: Inherit via internal rule
  Frame Conversion2 : FrameConversion  OutFrame=Sample-based
  Gain : Gain  Gain=1/2  SaturateOnIntegerOverflow=on  OutDataTypeStr=Inherit: Same as input  ParamDataTypeStr=Inherit: Same as input
  Math Function : Math  Operator=hermitian  SaturateOnIntegerOverflow=on
  Matrix Multiply : Product  Multiplication=Matrix(*)
  Matrix Multiply1 : Product  Multiplication=Matrix(*)
  Product : Product  Inputs=/*  SaturateOnIntegerOverflow=on  OutDataTypeStr=Inherit: Same as first input
  Product1 : Product  SaturateOnIntegerOverflow=on  OutDataTypeStr=Inherit: Same as first input
  Product2 : Product  Inputs=*/  SaturateOnIntegerOverflow=on  OutDataTypeStr=Inherit: Same as first input
  Signal Specification : SignalSpecification  Dimensions=[L,L]
  Stabilize : Subsystem
  Sum : Sum  SaturateOnIntegerOverflow=on  OutDataTypeStr=Inherit: Same as first input
  Sum1 : Sum  Inputs=+-|  SaturateOnIntegerOverflow=on
  Sum2 : Sum  Inputs=++|  SaturateOnIntegerOverflow=on
  conj : Math  Operator=conj  SaturateOnIntegerOverflow=on
  W(n) : Outport  InitialOutput=flipud(ic(:))
  wires:
  Constant/1 -> Sum/2
  conj/1 -> Product1/2
  [lambda] -> Product2/2
  Stabilize/1(Out) -> Product2/1
  Product2/1 -> Gain/1
  Lambda/1 -> [lambda]
  Gain/1 -> Signal Specification/1
  Correlation/1 -> Stabilize/1(In)  "P(n-1)"
  Reset/1 -> Correlation/2
  Signal Specification/1 -> Sum1/1, Matrix Multiply1/1
  Sum2/1 -> W(n)/1
  X/1 -> Dot Product/1, Matrix Multiply1/2
  Err/1 -> Product1/1
  W(n-1)/1 -> Sum2/1
  Product1/1 -> Sum2/2
  Sum1/1 -> Frame Conversion2/1
  Matrix Multiply/1 -> Sum1/2  "k(n)*X*(n-1)"
  Math Function/1 -> Matrix Multiply/2
  Product/1 -> Matrix Multiply/1, conj/1  "k(n)"
  Matrix Multiply1/1 -> Dot Product/2, Product/2, Math Function/1  "P(n-1)*X"
  Sum/1 -> Product/1
  Dot Product/1 -> Sum/1  "X'P(n-1).X)"
  Frame Conversion2/1 -> Correlation/1

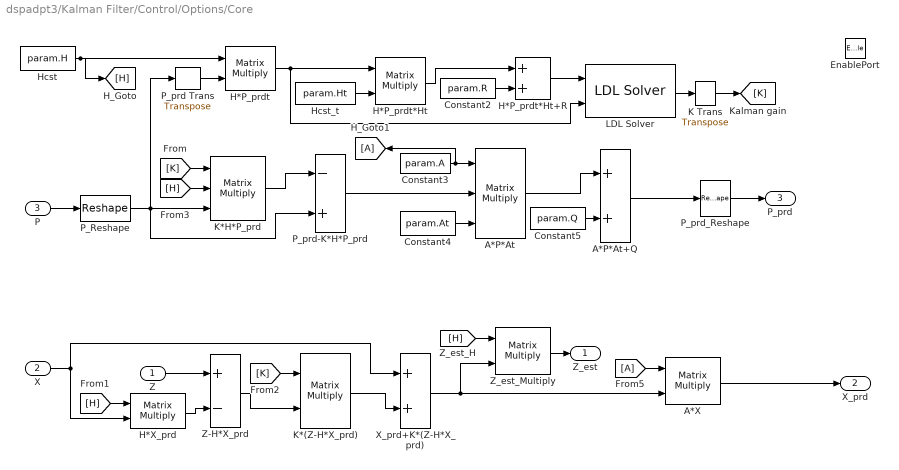
== system dspadpt3/Kalman Filter/Control/Options/Core ==
  Z : Inport
  X : Inport  Port=2
  P : Inport  Port=3
  EnablePort : EnablePort
  A*P*At : Product  Inputs=3  Multiplication=Matrix(*)  OutDataTypeStr=Inherit: Inherit via back propagation  InputSameDT=on
  A*P*At+Q : Sum  OutDataTypeStr=Inherit: Inherit via back propagation  InputSameDT=on
  A*X : Product  Multiplication=Matrix(*)  InputSameDT=on
  Constant2 : Constant  Value=param.R  VectorParams1D=off  OutDataTypeStr=Inherit: Inherit via back propagation
  Constant3 : Constant  Value=param.A  VectorParams1D=off  OutDataTypeStr=Inherit: Inherit via back propagation
  Constant4 : Constant  Value=param.At  VectorParams1D=off  OutDataTypeStr=Inherit: Inherit via back propagation
  Constant5 : Constant  Value=param.Q  VectorParams1D=off  OutDataTypeStr=Inherit: Inherit via back propagation
  H*P_prdt : Product  Multiplication=Matrix(*)  OutDataTypeStr=Inherit: Inherit via back propagation  InputSameDT=on
  H*P_prdt*Ht : Product  Multiplication=Matrix(*)  OutDataTypeStr=Inherit: Inherit via back propagation  InputSameDT=on
  H*P_prdt*Ht+R : Sum  OutDataTypeStr=Inherit: Inherit via back propagation  InputSameDT=on
  H*X_prd : Product  Multiplication=Matrix(*)  OutDataTypeStr=Inherit: Inherit via back propagation  InputSameDT=on
  Hcst : Constant  Value=param.H  VectorParams1D=off  OutDataTypeStr=Inherit: Inherit via back propagation
  Hcst_t : Constant  Value=param.Ht  VectorParams1D=off  OutDataTypeStr=Inherit: Inherit via back propagation
  K Trans : dspmtrx3/Transpose  SystemSampleTime=-1  Hermitian=off  overflowFlag=off
  K*(Z-H*X_prd) : Product  Multiplication=Matrix(*)  InputSameDT=on
  K*H*P_prd : Product  Inputs=3  Multiplication=Matrix(*)  InputSameDT=on  OutDataTypeStr=Inherit: Same as first input
  LDL Solver : dspsolvers/LDL Solver  SystemSampleTime=-1  errmode=Warning
      settings: RTWMemSecFuncInitTerm=Default  RTWMemSecFuncExecute=Default  RTWMemSecDataConstants=Default  RTWMemSecDataInternal=Default  RTWMemSecDataParameters=Default
  P_Reshape : Reshape  OutputDimensionality=Customize  OutputDimensions=[len_state, len_state]
  P_prd Trans : dspmtrx3/Transpose  SystemSampleTime=-1  Hermitian=off  overflowFlag=off
  P_prd-K*H*P_prd : Sum  Inputs=-+  OutDataTypeStr=Inherit: Inherit via back propagation  InputSameDT=on
  P_prd_Reshape : Reshape  OutputDimensionality=Column vector (2-D)
  X_prd+K*(Z-H*X_prd) : Sum  InputSameDT=on
  Z-H*X_prd : Sum  Inputs=+-  InputSameDT=on  OutDataTypeStr=Inherit: Same as first input
  Z_est_Multiply : Product  Multiplication=Matrix(*)  InputSameDT=on
  Z_est : Outport
  X_prd : Outport  Port=2
  P_prd : Outport  Port=3
  wires:
  A*X/1 -> X_prd/1
  A*P*At+Q/1 -> P_prd_Reshape/1
  P_prd-K*H*P_prd/1 -> A*P*At/2
  X/1 -> X_prd+K*(Z-H*X_prd)/1, H*X_prd/2
  P/1 -> P_Reshape/1
  Z-H*X_prd/1 -> K*(Z-H*X_prd)/2
  K*(Z-H*X_prd)/1 -> X_prd+K*(Z-H*X_prd)/2
  H*X_prd/1 -> Z-H*X_prd/2
  [K] -> K*H*P_prd/1
  [H] -> K*H*P_prd/2
  K*H*P_prd/1 -> P_prd-K*H*P_prd/1
  A*P*At/1 -> A*P*At+Q/1
  Constant5/1 -> A*P*At+Q/2
  Constant4/1 -> A*P*At/3
  Constant2/1 -> H*P_prdt*Ht+R/2
  H*P_prdt*Ht/1 -> H*P_prdt*Ht+R/1
  Z/1 -> Z-H*X_prd/1
  [K] -> K*(Z-H*X_prd)/1
  [H] -> H*X_prd/1
  K Trans/1 -> [K]
  P_prd Trans/1 -> H*P_prdt/2
  H*P_prdt/1 -> LDL Solver/2, H*P_prdt*Ht/1
  H*P_prdt*Ht+R/1 -> LDL Solver/1
  LDL Solver/1 -> K Trans/1
  P_prd_Reshape/1 -> P_prd/1
  [H] -> Z_est_Multiply/1
  Z_est_Multiply/1 -> Z_est/1
  X_prd+K*(Z-H*X_prd)/1 -> A*X/2, Z_est_Multiply/2
  [A] -> A*X/1
  Constant3/1 -> A*P*At/1, [A]
  P_Reshape/1 -> K*H*P_prd/3, P_prd-K*H*P_prd/2, P_prd Trans/1
  Hcst/1 -> [H], H*P_prdt/1
  Hcst_t/1 -> H*P_prdt*Ht/2

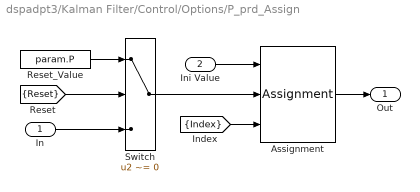
== system dspadpt3/Kalman Filter/Control/Options/P_prd_Assign ==
  In : Inport
  Ini Value : Inport  Port=2
  Assignment : Assignment  NumberOfDimensions=2  IndexOptions=Assign all,Index vector (port)  Indices=-1,1  OutputSizes=slselsubs([num_rows, num_cols],1),slselsubs([num_rows, num_cols],2)
  Reset_Value : Constant  Value=param.P  VectorParams1D=off  OutDataTypeStr=Inherit: Inherit via back propagation
  Switch : Switch  Criteria=u2 ~= 0  SaturateOnIntegerOverflow=on  InputSameDT=on
  Out : Outport
  wires:
  [Index] -> Assignment/3
  Ini Value/1 -> Assignment/1
  Assignment/1 -> Out/1
  Reset_Value/1 -> Switch/1
  [Reset] -> Switch/2
  In/1 -> Switch/3
  Switch/1 -> Assignment/2

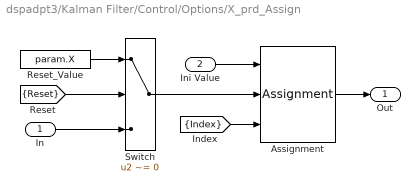
== system dspadpt3/Kalman Filter/Control/Options/X_prd_Assign ==
  In : Inport
  Ini Value : Inport  Port=2
  Assignment : Assignment  NumberOfDimensions=2  IndexOptions=Assign all,Index vector (port)  Indices=-1,1  OutputSizes=slselsubs([num_rows, num_cols],1),slselsubs([num_rows, num_cols],2)
  Reset_Value : Constant  Value=param.X  VectorParams1D=off  OutDataTypeStr=Inherit: Inherit via back propagation
  Switch : Switch  Criteria=u2 ~= 0  SaturateOnIntegerOverflow=on  InputSameDT=on
  Out : Outport
  wires:
  Assignment/1 -> Out/1
  Ini Value/1 -> Assignment/1
  [Index] -> Assignment/3
  Reset_Value/1 -> Switch/1
  [Reset] -> Switch/2
  In/1 -> Switch/3
  Switch/1 -> Assignment/2

== system dspadpt3/Kalman Filter/Control/Options/Z_est_Assign ==
  In : Inport
  Assignment : Assignment  NumberOfDimensions=2  OutputInitialize=Specify size for each dimension in table  IndexOptions=Assign all,Index vector (port)  Indices=-1,1  OutputSizes=slselsubs([num_rows, num_cols],1),slselsubs([num_rows, num_cols],2)
  Reset_Value : Constant  Value=reset_value  VectorParams1D=off  OutDataTypeStr=Inherit: Inherit via back propagation
  Switch : Switch  Criteria=u2 ~= 0  SaturateOnIntegerOverflow=on  InputSameDT=on
  Out : Outport
  wires:
  [Index] -> Assignment/2
  Assignment/1 -> Out/1
  Reset_Value/1 -> Switch/1
  [Reset] -> Switch/2
  In/1 -> Switch/3
  Switch/1 -> Assignment/1

== system dspadpt3/RLS Filter/Frame-Based RLS Filter/Update/Stabilize ==
  In : Inport
  Sum2 : Sum  Inputs=|++  SaturateOnIntegerOverflow=on  InputSameDT=on  OutDataTypeStr=Inherit: Same as first input
  conj1 : Math  Operator=hermitian  SaturateOnIntegerOverflow=on
  Out : Outport
  wires:
  Sum2/1 -> Out/1
  conj1/1 -> Sum2/1
  In/1 -> Sum2/2, conj1/1  "P(n-1)/Lambda"
